simulink model "xEMU_SimulationModel3_rule1"  (R2017b)
settings: Solver=ode4  StartTime=0.0  StopTime=8192  FixedStep=0.01  RelTol=1e-3
undefined symbols (not defined in the file): a1, a2, a3, a4, ACO, BAT, Battery, DCT, DRT, EMS, ENV, Fahrzyklus_VS_modell, height_BAT, leistung, lib_bat, Maximum, Maximum_position, Num_cells, P_FC_max_long, P_FC_min_long, P_FC_step_max, Pbat_charge_max, Pbat_discharge_max, Pfc_max, Pfc_min, SOC_tar, time_peaks, TRM, velocity_peaks
libraries: simulink x5
(part 12 of 15)

== system xEMU_SimulationModel3_rule1/Battery (BAT)_mittel/Subsystem1/ElectricalCircuit/Cellelement_Elem1/VoltageSource_Elem7 ==
  T : Inport
  SoC : Inport  Port=2
  Object : Lookup_n-D  BreakpointsForDimension1=[10 25 35 45]  BreakpointsForDimension2=[0 0.1 0.2 0.3 0.4 0.5 0.6 0.7 0.8 0.9 1 1.1 1.2 1.3 1.4 1.5 1.6 1.7 1.8 1.9 2 2.1 2.2 2.3 2.4 2.5 2.6 2.7 2.8 2.9 3 3.1 3.2 3.3 3.4 3.5 3.6 3.7 3.8 3.9 4 4.1 4.2 4.3 4.4 4.5 4.6 4.7 4.8 4.9 5 5.1 5.2 5.3 5.4 5.5 5.6 5.7 5.8 5.9 6 6.1 6.2 6.3 6.4 6.5 6.6 6.7 6.8 6.9 7 7.1 7.2 7.3 7.4 7.5 7.6 7.7 7.8 7.9 8 8.1 8.2 8.3 8.4 8.5 8.6 8.7 8.8 8.9 9 9.1 9.2 9.3 9.4 9.5 9.6 9.7 9.8 9.9 10 10.1 10.2 10.3 10.4 10.5 10.6 10.7 10.8 10.9 11 11.1 11.2 11.3 11.4 11.5 11.6 11.7 11.8 11.9 12 12.1 12.2 12.3 12.4 12.5 12.6 12.7 12.8 12.9 13 13.1 13.2 13.3 13.4 13.5 13.6 13.7 13.8 13.9 14 14.1 14.2 14.3 14.4 14.5 14.6 14.7 14.8 14.9 15 15.1 15.2 15.3 15.4 15.5 15.6 15.7 15.8 15.9 16 16.1 16.2 16.3 16.4 16.5 16.6 16.7 16.8 16.9 17 17.1 17.2 17.3 17.4 17.5 17.6 17.7 17.8 17.9 18 18.1 18.2 18.3 18.4 18.5 18.6 18.7 18.8 18.9 19 19.1 19.2 19.3 19.4 19.5 19.6 19.7 19.8 19.9 20 20.1 20.2 20.3 20.4 20.5 20.6 20.7 20.8 20.9 21 21.1 21.2 21.3 21.4 21.5 21.6 21.7 21.8 21.9 22 22.1 22.2 22.3 22.4 22.5 22.6 22.7 22.8 22.9 23 23.1 23.2 23.3 23.4 23.5 23.6 23.7 23.8 23.9 24 24.1 24.2 24.3 24.4 24.5 24.6 24.7 24.8 24.9 25 25.1 25.2 25.3 25.4 25.5 25.6 25.7 25.8 25.9 26 26.1 26.2 26.3 26.4 26.5 26.6 26.7 26.8 26.9 27 27.1 27.2 27.3 27.4 27.5 27.6 27.7 27.8 27.9 28 28.1 28.2 28.3 28.4 28.5 28.6 28.7 28.8 28.9 29 29.1 29.2 29.3 29.4 29.5 29.6 29.7 29.8 29.9 30 30.1 30.2 30.3 30.4 30.5 30.6 30.7 30.8 30.9 31 31.1 31.2 31.3 31.4 31.5 31.6 31.7 31.8 31.9 32 32.1 32.2 32.3 32.4 32.5 32.6 32.7 32.8 32.9 33 33.1 33.2 33.3 33.4 33.5 33.6 33.7 33.8 33.9 34 34.1 34.2 34.3 34.4 34.5 34.6 34.7 34.8 34.9 35 35.1 35.2 35.3 35.4 35.5 35.6 35.7 35.8 35.9 36 36.1 36.2 36.3 36.4 36.5 36.6 36.7 36.8 36.9 37 37.1 37.2 37.3 37.4 37.5 37.6 37.7 37.8 37.9 38 38.1 38.2 38.3 38.4 38.5 38.6 38.7 38.8 38.9 39 39.1 39.2 39.3 39.4 39.5 39.6 39.7 39.8 39.9 40 40.1 40.2 40.3 40.4 40.5 40.6 40.7 40.8 40.9 41 41.1 41.2 41.3 41.4 41.5 41.6 41.7 41.8 41.9 42 42.1 42.2 42.3 42.4 42.5 42.6 42.7 42.8 42.9 43 43.1 43.2 43.3 43.4 43.5 43.6 43.7 43.8 43.9 44 44.1 44.2 44.3 44.4 44.5 44.6 44.7 44.8 44.9 45 45.1 45.2 45.3 45.4 45.5 45.6 45.7 45.8 45.9 46 46.1 46.2 46.3 46.4 46.5 46.6 46.7 46.8 46.9 47 47.1 47.2 47.3 47.4 47.5 47.6 47.7 47.8 47.9 48 48.1 48.2 48.3 48.4 48.5 48.6 48.7 48.8 48.9 49 49.1 49.2 49.3 49.4 49.5 49.6 49.7 49.8 49.9 50 50.1 50.2 50.3 50.4 50.5 50.6 50.7 50.8 50.9 51 51.1 51.2 51.3 51.4 51.5 51.6 51.7 51.8 51.9 52 52.1 52.2 52.3 52.4 52.5 52.6 52.7 52.8 52.9 53 53.1 53.2 53.3 53.4 53.5 53.6 53.7 53.8 53.9 54 54.1 54.2 54.3 54.4 54.5 54.6 54.7 54.8 54.9 55 55.1 55.2 55.3 55.4 55.5 55.6 55.7 55.8 55.9 56 56.1 56.2 56.3 56.4 56.5 56.6 56.7 56.8 56.9 57 57.1 57.2 57.3 57.4 57.5 57.6 57.7 57.8 57.9 58 58.1 58.2 58.3 58.4 58.5 58.6 58.7 58.8 58.9 59 59.1 59.2 59.3 59.4 59.5 59.6 59.7 59.8 59.9 60 60.1 60.2 60.3 60.4 60.5 60.6 60.7 60.8 60.9 61 61.1 61.2 61.3 61.4 61.5 61.6 61.7 61.8 61.9 62 62.1 62.2 62.3 62.4 62.5 62.6 62.7 62.8 62.9 63 63.1 63.2 63.3 63.4 63.5 63.6 63.7 63.8 63.9 64 64.1 64.2 64.3 64.4 64.5 64.6 64.7 64.8 64.9 65 65.1 65.2 65.3 65.4 65.5 65.6 65.7 65.8 65.9 66 66.1 66.2 66.3 66.4 66.5 66.6 66.7 66.8 66.9 67 67.1 67.2 67.3 67.4 67.5 67.6 67.7 67.8 67.9 68 68.1 68.2 68.3 68.4 68.5 68.6 68.7 68.8 68.9 69 69.1 69.2 69.3 69.4 69.5 69.6 69.7 69.8 69.9 70 70.1 70.2 70.3 70.4 70.5 70.6 70.7 70.8 70.9 71 71.1 71.2 71.3 71.4 71.5 71.6 71.7 71.8 71.9 72 72.1 72.2 72.3 72.4 72.5 72.6 72.7 72.8 72.9 73 73.1 73.2 73.3 73.4 73.5 73.6 73.7 73.8 73.9 74 74.1 74.2 74.3 74.4 74.5 74.6 74.7 74.8 74.9 75 75.1 75.2 75.3 75.4 75.5 75.6 75.7 75.8 75.9 76 76.1 76.2 76.3 76.4 76.5 76.6 76.7 76.8 76.9 77 77.1 77.2 77.3 77.4 77.5 77.6 77.7 77.8 77.9 78 78.1 78.2 78.3 78.4 78.5 78.6 78.7 78.8 78.9 79 79.1 79.2 79.3 79.4 79.5 79.6 79.7 79.8 79.9 80 80.1 80.2 80.3 80.4 80.5 80.6 80.7 80.8 80.9 81 81.1 81.2 81.3 81.4 81.5 81.6 81.7 81.8 81.9 82 82.1 82.2 82.3 82.4 82.5 82.6 82.7 82.8 82.9 83 83.1 83.2 83.3 83.4 83.5 83.6 83.7 83.8 83.9 84 84.1 84.2 84.3 84.4 84.5 84.6 84.7 84.8 84.9 85 85.1 85.2 85.3 ...(+706 chars)]  Table=[2.06325426332686 2.06399433941078 2.06488931344211 2.0657018181389 2.0664803797572 2.06736288637271 2.06807144607228 2.06883571716219 2.06952595426618 2.07025915765007 2.07095524992837 2.0716614781761 2.07234743039771 2.07304352267784 2.07370631481565 2.07442667845301 2.07513179542366 2.07572844478091 2.07632509413634 2.07702118232373 2.07768118378557 2.07821448103641 2.07881113039002 2.07940777974727 2.08010386793285 2.0807005172901 2.08119772372629 2.08179437308354 2.08239102243897 2.08294743640934 2.08348487822695 2.0840815275842 2.0847765007496 2.08527482220234 2.08587147155777 2.08636867799214 2.08696532734757 2.08746253378013 2.08796050621806 2.0885167436275 2.08905796478586 2.08965024126337 2.09005148346185 2.09064465412848 2.09114186056104 2.09163906699541 2.09223571635084 2.09273292278522 2.09323012921595 2.09372733564851 2.09422454208107 2.0947217485118 2.09521895494618 2.09571616137691 2.09621336781129 2.09671057424202 2.0972077806764 2.09760554418608 2.09810275061864 2.09859995705119 2.09909716348193 2.09959436991448 2.09999213342235 2.10048933985672 2.10098654628746 2.10148375272183 2.1018815162297 2.10237872266407 2.10286848779969 2.10327369260631 2.10377089903704 2.10418373194731 2.10476530780943 2.10517250756716 2.10566027774985 2.1061574841824 2.10645580886012 2.10695301529267 2.10745022172523 2.10792491641664 2.10834519166747 2.10874295517533 2.10924016160789 2.10963792511575 2.11013513155012 2.11053289505617 2.11103010149054 2.1114278649984 2.11182562850809 2.11232283494064 2.1127205984485 2.11311836195819 2.11357839550814 2.11401333190224 2.11441109541011 2.11490830184266 2.11530606535052 2.11573870468929 2.11620103529094 2.11659879880062 2.11709600523318 2.11759320757301 2.11799097108087 2.11845099004869 2.11888594102129 2.11928370453097 2.11968146803883 2.12017867447321 2.12057643798107 2.12094270803892 2.12127252616847 2.12167028967633 2.12216749610889 2.12256525961675 2.12296302312643 2.12336078663429 2.12375855014398 2.12418343651453 2.12455408125243 2.12495184476211 2.12534960826997 2.12574737178147 2.12614513529115 2.12654289879902 2.1269406623087 2.12736724570825 2.12783563225094 2.12823339575698 2.128571665593 2.12902892277452 2.12938548939324 2.12982444979207 2.13026408722299 2.13071941973431 2.13101774441202 2.13147588758996 2.13181327142956 2.13221103493925 2.13260879844711 2.13300656195679 2.13340432546465 2.13370265014237 2.13410041365205 2.13449817715809 2.13489594066778 2.13529370417564 2.13569146768532 2.13608923119318 2.13648699470286 2.13678531938058 2.13718308288844 2.13758084639812 2.13797860990781 2.13832554235321 2.13866087738688 2.13897301868201 2.13937078219169 2.13966910686941 2.14006687037727 2.14046463388513 2.14086239739299 2.14126016090268 2.14165792441054 2.14205568792022 2.14235401259793 2.14275177610762 2.14314953961548 2.14354730312334 2.14388762424526 2.14424339131074 2.14464115482042 2.14503891832828 2.1452967874573 2.14563556359281 2.14603332710067 2.14633164768566 2.14672941119352 2.14702773587123 2.14742549938092 2.14782326288878 2.14802214464362 2.14841990815148 2.14881767166116 2.14911599633888 2.14951375984674 2.14981208043355 2.15011040511308 2.15050816862095 2.15090593213063 2.15110481388365 2.15150257739333 2.15190034090119 2.15219942862393 2.15249698616753 2.15289474967358 2.15329251318326 2.15359083786097 2.15398860136884 2.15431605674633 2.15458524663336 2.15498301014122 2.15528133482076 2.15567909832862 2.15597741891361 2.15634803031096 2.15667350709919 2.15697182768599 2.15736959119386 2.15774254543299 2.15796623645656 2.15836399996442 2.15875141051424 2.15896064522713 2.15935840873681 2.15965673341452 2.15995505399951 2.16025337867723 2.16065114218691 2.16094946277008 2.16124778744961 2.16164555095747 2.16192421241581 2.162242196222 2.16254051680517 2.16283884148652 2.16320058224773 2.16343548674922 2.1638332502589 2.16413157493662 2.16442989551979 2.16472822019932 2.16511214652138 2.16532486546203 2.16572262897171 2.16592151072655 2.16631927423441 ...(+63680 chars)]  ExtrapMethod=Clip  RndMeth=Simplest  InputSameDT=on
  tag scope: ID7_ObjV=global
  wires:
  Object/1 -> [ID7_ObjV]
  T/1 -> Object/1
  SoC/1 -> Object/2
